simulink model "AUV_model"  (R2022a)
settings: Solver=VariableStepAuto  StartTime=0.0  StopTime=25  FixedStep=1e-4  RelTol=1e-3
values from neighbouring files (symbols this model uses):
  Ixx = 1467656.991	Ixy = 5625.578	Ixz = -59590.923    [Parameters.m]
  Iyy = 1.4676    [Parameters.m]
  Izz = 2.4720    (= 2.472)    [Parameters.m]
  m = 32.135    [Parameters.m]
libraries: slpidlib x24
(part 3 of 3)

== matlab function AUV_model/MATLAB Function ==
  data: t input; x_d output; y_d output; z_d output
function [x_d, y_d, z_d] = fcn(t)
%%  螺旋轨迹
    % 定义基础半径随时间变化
    r = 0.1 * t; % 半径从0逐渐增加，每秒增加0.1单位

    % 计算轨迹
    x_d = r .* sin(0.5 * t); % X 方向，半径与时间相关
    y_d = r .* cos(0.5 * t);  % Y 方向，半径与时间相关
    z_d = 0.5 * t;                  % Z 方向，线性上升


%%  0-5秒在z_d等于0的平面，进行2*2的正方形顺时针运动，5-10在z_d等于2的平面，进行2*2的正方形顺时针运动
% 初始化
%     side_length = 2;  % 正方形边长
%     z1 = 0;  % 第一段的z值
%     z2 = 2;  % 第二段的z值
% 
%     % 0-5秒：在 z = 0 平面上顺时针运动
%     if t >= 0 && t < 5
%         % 映射时间到正方形路径的四个顶点
%         time_step = mod(t, 1);  % 每秒内的时间位置，周期为1秒
%         if time_step < 0.25
%             x_d = time_step * side_length;
%             y_d = 0;
%         elseif time_step < 0.5
%             x_d = side_length;
%             y_d = (time_step - 0.25) * side_length;
%         elseif time_step < 0.75
%             x_d = side_length - (time_step - 0.5) * side_length;
%             y_d = side_length;
%         else
%             x_d = 0;
%             y_d = side_length - (time_step - 0.75) * side_length;
%         end
%         z_d = z1;  % 在平面 z = 0 上
% 
%     % 5-10秒：在 z = 2 平面上顺时针运动
%     elseif t >= 5 && t < 10
%         % 映射时间到正方形路径的四个顶点
%         time_step = mod(t - 5, 1);  % 每秒内的时间位置，周期为1秒
%         if time_step < 0.25
%             x_d = time_step * side_length;
%             y_d = 0;
%         elseif time_step < 0.5
%             x_d = side_length;
%             y_d = (time_step - 0.25) * side_length;
%         elseif time_step < 0.75
%             x_d = side_length - (time_step - 0.5) * side_length;
%             y_d = side_length;
%         else
%             x_d = 0;
%             y_d = side_length - (time_step - 0.75) * side_length;
%         end
%         z_d = z2;  % 在平面 z = 2 上

%%  
%     % 正方形边长
%     side_length = 5;  
% 
%     % 设定不同的平面
%     z_planes = [0, 3, 6, 9];
%     
%     % 每个平面上的周期，正方形的运动完成一圈需要的时间
%     period = 5;  
% 
%     % 计算当前平面，t / period 即计算完成了多少圈
%     plane_index = mod(floor(t / period), length(z_planes)) + 1;  % 使用mod来切换平面
%     z_d = z_planes(plane_index);  % 获取当前平面的z值
% 
%     % 计算每个平面内的顺时针正方形运动
%     time_step = mod(t, period);  % 在每个平面内的时间位置，周期为5秒
%     time_step = time_step / period;  % 归一化到[0,1]之间
% 
%     % 根据time_step计算四个顶点的坐标
%     if time_step < 0.25
%         x_d = time_step * side_length;
%         y_d = 0;
%     elseif time_step < 0.5
%         x_d = side_length;
%         y_d = (time_step - 0.25) * side_length;
%     elseif time_step < 0.75
%         x_d = side_length - (time_step - 0.5) * side_length;
%         y_d = side_length;
%     else
%         x_d = 0;
%         y_d = side_length - (time_step - 0.75) * side_length;
%     end

end

== matlab function AUV_model/逆变换phi/MATLAB Function ==
  data: u_x input; tao_x output; u_y input; u_z input; tao_y output; tao_z output; phi_rad_d output
function [tao_x, tao_y, tao_z,phi_rad_d] = Inverse_transformation(u_x, u_y, u_z)
    % 逆变换 通过惯性坐标系虚拟力 ux, uy, uz 期望 psi_d 算出运动坐标系的 tao_x, tao_y, tao_z

    % 输入值
    %u_x = 150;
    %u_y = 100;
    %psi_cur = pi/3; % 当前航向角
    
    % 求解
    phi_rad_d=-atan2(u_y,u_z);
    tao_x=u_x;
    tao_z = u_z/cos(phi_rad_d);
    tao_y=-1*tao_z*sin(phi_rad_d);
    
    %fprintf('tao_x = %.4f, tao_y = %.4f, psi_d = %.4f  %.4f\n', tao_x, tao_y, psi_rad_d,psi_rad_d*180/pi);
end

== matlab function AUV_model/Subsystem/位置动力学/MATLAB Function ==
  data: tao_x input; u_dot output; tao_y input; tao_z input; p input; q input; v_dot output; w_dot output; r input; u input; v input; w input; m input
function [u_dot,v_dot,w_dot] = pos_dyna(tao_x,tao_y,tao_z,p,q,r,u,v,w,m)
%假设Zg=0
%u_dot = tao_x/m + u*r - w*q;
%v_dot = tao_y/m + w*p - u*r;
%w_dot = tao_z/m + u*q - v*p;


u_dot = tao_x/m ;
v_dot = tao_y/m ;
w_dot = tao_z/m ;
end

== matlab function AUV_model/Subsystem/姿态运动学/MATLAB Function ==
  data: wbx input; roll_dot output; wby input; wbz input; pitch input; roll input; pitch_dot output; yaw_dot output
function [roll_dot,pitch_dot,yaw_dot] = att_kine(wbx,wby,wbz,pitch,roll)
%姿态运动学  从运动坐标系变换到固定坐标系
roll_dot = wbx + tan(pitch)*sin(roll)*wby + tan(pitch)*cos(roll)*wbz;
pitch_dot = cos(roll)*wby - sin(roll)*wbz;
yaw_dot = (sin(roll)/cos(pitch))*wby + (cos(roll)/cos(pitch))*wbz;
end

== matlab function AUV_model/Subsystem/姿态动力学/MATLAB Function ==
  data: tao_k input; tao_m input; tao_n input; p input; q input; r input; Ixx input; p_dot output; Iyy input; Izz input; q_dot output; r_dot output
function [p_dot,q_dot,r_dot] = pos_dyna(tao_k,tao_m,tao_n,p,q,r,Ixx,Iyy,Izz)
%假设Zg=0
%p_dot = (tao_k - (Izz-Iyy)*q*r)/Ixx;
%q_dot = (tao_m - (Ixx-Izz)*r*q)/Iyy;
%r_dot = (tao_n - (Iyy-Ixx)*p*q)/Izz;

p_dot = (tao_k)/Ixx;
q_dot = (tao_m)/Iyy;
r_dot = (tao_n)/Izz;


end

== matlab function AUV_model/Subsystem/位置运动学/MATLAB Function ==
  data: u input; ue output; v input; w input; ve output; we output; roll input; pitch input; yaw input
function [ue,ve,we] = pos_kine(u,v,w,roll,pitch,yaw)  %roll fai pitch sita yaw pusi
%位置运动学  从运动坐标系变换到固定坐标系
%ue = cos(yaw)*cos(pitch)*u+(cos(yaw)*sin(pitch)*sin(roll)-sin(yaw)*cos(roll))*v+(cos(yaw)*sin(pitch)*cos(roll)+sin(yaw)*sin(roll)*w);
%ve = sin(yaw)*cos(pitch)*u+(sin(yaw)*sin(pitch)*sin(roll)+cos(yaw)*cos(roll))*v+(sin(yaw)*sin(pitch)*cos(roll)-cos(yaw)*sin(roll)*w);
%we = -sin(pitch)*u+cos(pitch)*sin(roll)*v+cos(pitch)*cos(roll)*w;

ue = u;
ve = v;
we = w;
end

== matlab function AUV_model/模型/位置动力学/MATLAB Function ==
  data: tao_x input; u_dot output; tao_y input; tao_z input; p input; q input; v_dot output; w_dot output; r input; u input; v input; w input; m input
function [u_dot,v_dot,w_dot] = pos_dyna(tao_x,tao_y,tao_z,p,q,r,u,v,w,m)
%假设Zg=0
%u_dot = tao_x/m + u*r - w*q;
%v_dot = tao_y/m + w*p - u*r;
%w_dot = tao_z/m + u*q - v*p;


u_dot = tao_x/m ;
v_dot = tao_y/m ;
w_dot = tao_z/m ;
end
